simulink model "PVtestsiteeight"  (Simulink 10.1)
settings: Solver=FixedStepDiscrete  StartTime=0.0  StopTime=inf  FixedStep=Ts  RelTol=1e-3
PreLoadFcn:
  | init_DCDCDCAC_new
InitFcn:
  | init_DCDCDCAC_new
undefined symbols (not defined in the file or in its folder): D1, Delta, I, Left, Right, type, V
libraries: powerlib x174, powerlib_meascontrol x3, ssn_lib x2, artemis x1
(part 1 of 3)
settings Model: ARTEMISmethode_block_infos=$$__separator__$$PVtestsiteeight/SS_Grid/ARTEMIS Guide$$__separator__$$  Creator=jz38692  LastModifiedBy=jz38692
settings DataIOCC: ExternalInput=ILreplay  SaveFormat=Dataset  SaveOutput=off  SignalLogging=off  DSMLogging=off  SaveTime=off  DSMLoggingName=signal_recordone
settings OptimizationCC: LifeSpan=auto
settings DebuggingCC: UnderspecifiedInitializationDetection=Simplified  MergeDetectMultiDrivingBlocksExec=error  SFUnexpectedBacktrackingDiag=error  SFNoUnconditionalDefaultTransitionDiag=error  SFExecutionAtInitializationDiag=warning
settings HardwareCC: ProdBitPerPointer=64  ProdBitPerSizeT=64  ProdBitPerPtrDiffT=64  ProdLargestAtomicFloat=Float  ProdIntDivRoundTo=Zero  ProdEndianess=LittleEndian  ProdWordSize=64  ProdHWDeviceType=Intel->x86-64 (Windows64)
settings ModelReferenceCC: PropagateSignalLabelsOutOfModel=on
settings SFSimCC: SimUseLocalCustomCode=on
settings RTWCC: RTWUseLocalCustomCode=on
settings GRTTargetCC: TargetLangStandard=C99 (ISO)  CombineOutputUpdateFcns=on  GRTInterface=off
settings ConfigComp: CovMetricSettings=dwe  CovHtmlReporting=off  CovSaveCumulativeToWorkspaceVar=off  CovSaveSingleToWorkspaceVar=off  CovExternalEMLEnable=on
settings SimscapeCC: SimscapeNormalizeSystem=off

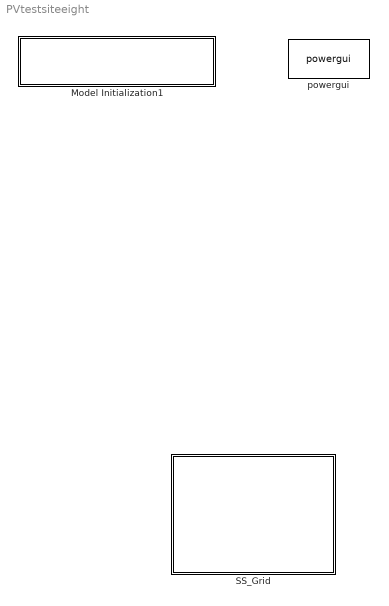
== system PVtestsiteeight ==
  Model Initialization1 : Subsystem  AncestorBlock=artemis/Tools /Misc/Model Initialization  mask(Model Functions){InitFcnX=init_DCDCDCAC_new, prel=on, posl=off, inif=on, strf=off}
      mask prompts: InitFcnX "Initialisation"; prel "Preload Function"; posl "PostLoad Function"; inif "InitFcn"; strf "StartFcn"
      mask init:
      | currentBlock = gcb;
      | root = bdroot(currentBlock);
      | 
      | if ~strcmp(get_param(root,'BlockDiagramType'),'library')
      |     if prel==1
      |         set_param(root, 'PreLoadFcn', InitFcnX);
      |     else
      |         set_param(root, 'PreLoadFcn', '');
      |     end
      |     if inif==1
      |         set_param(root, 'InitFcn', InitFcnX);
      |     else
      |         set_param(root, 'InitFcn', '');
      |     end
      |     if strf==1
      |         set_param(root, 'StartFcn', InitFcnX);
      |     else
      |         set_param(root, 'StartFcn', '');
      |     end
      |     if posl==1
      |         set_param(root, 'PostLoadFcn', InitFcnX);
      |     else
      |         set_param(root, 'PostLoadFcn', '');
      |     end
      | end
      | 
      | pos = get_param(currentBlock, 'Position');
      | width = pos(3) - pos(1); height = pos(4) - pos(2);
      | txt = [ upper(root) '\n' '- InitFcn. . . . . '  get_param(root, 'InitFcn') ];
      settings: CopyFcn=set_param(gcb,'LinkStatus','inactive')
      mask Display: text(5, height*0.5, txt, 'horizontalAlignment', 'left', 'verticalAlignment', 'middle') ;
  SS_Grid : Subsystem
  powergui : powerlib/powergui  Priority=1  SimulationMode=Discrete  SampleTime=5e-5  frequency=60  Iterations=50  frequencyindice=0  Pbase=100e6  ErrMax=1e-4  UnitsV=kV  UnitsW=MW  buscounter=0  FunctionMessages=off  echomessages=off  EnableUseOfTLC=off  CurrentSourceSwitches=off  DisableSnubberDevices=off  DisableRonSwitches=off  DisableVfSwitches=off  DisplayEquations=off  AutomaticDiscreteSolvers=off  SolverType=Backward Euler  Interpol=off  ExternalGateDelay=off  methode=off  Ts=100  x0status=blocks  SPID=off  SwTol=0  HookPort=off  NonlinearTolerance=1e-4  nMaxIteration=100  ContinueOnMaxIteration=off  RestoreLinks=warning  ResistiveCurrentMeasurement=off  Frange=[0:2:500]  Ylog=off  Xlog=on  ShowGrid=off  save=off  variable=ZData  structure=UIC  ZoomFFT=off  StartTime=1  cycles=50  DisplayStyle=1  fundamental=60  FreqAxis=off  MaxFrequency=10000  frequencyindicesteady=1  RmsSteady=1  display=off

== system PVtestsiteeight/Model Initialization1 ==

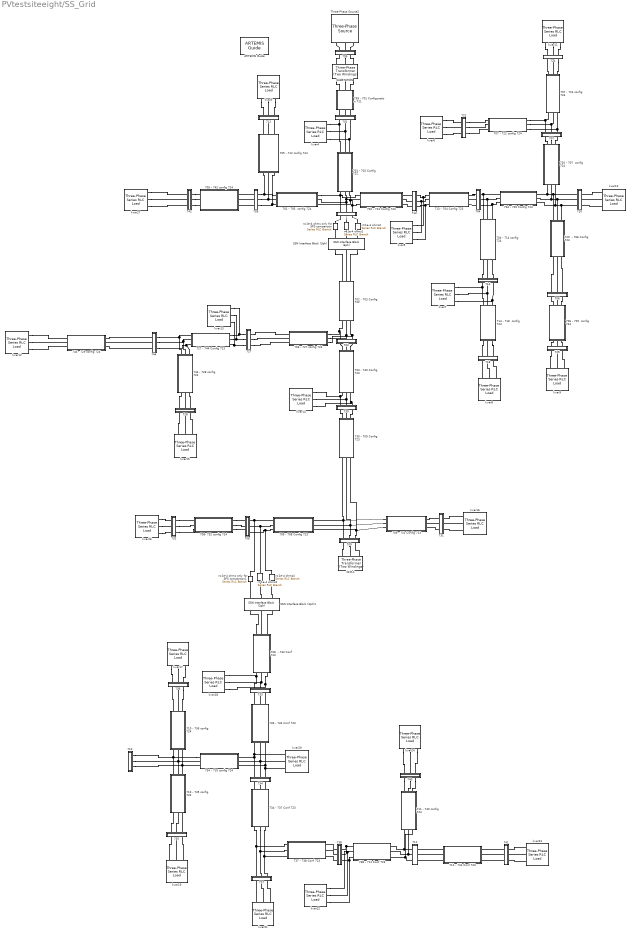
== system PVtestsiteeight/SS_Grid ==
  " 738 - 711 Conf 723 " : Subsystem  mask{D=0.1219}
      mask prompts: D "Distance (km)"
   kvar{5..11,14,16..24,26..27} (19 alike) : powerlib/Elements/Three-Phase Series RLC Load  LConnTagsString=A|B|C  Configuration=Y (grounded)  NominalVoltage=4800  Vabc=[4.8e3 4.8e3 4.8e3]/sqrt(3)  Vabcp=[1e3 1e3 1e3]  NominalFrequency=60  UnbalancedPower=on  ActivePower=10000  InductivePower=0  CapacitivePower=0  Pabc=[10e3 10e3 10e3]  QLabc=[0 0 0]  QCabc=[0 0 0]  Pabcp=[10e3 9e3 11e3]  QLabcp=[100 90 110]  QCabcp=[100 90 110]  Measurements=None  LoadType=constant Z
  " kvar12" : powerlib/Elements/Three-Phase Series RLC Load  LConnTagsString=A|B|C  Configuration=Y (grounded)  NominalVoltage=4800  Vabc=[4.8e3 4.8e3 4.8e3]/sqrt(3)  Vabcp=[1e3 1e3 1e3]  NominalFrequency=60  UnbalancedPower=off  ActivePower=100000  InductivePower=5000  CapacitivePower=0  Pabc=[10e3 10e3 10e3]  QLabc=[0 0 0]  QCabc=[0 0 0]  Pabcp=[10e3 9e3 11e3]  QLabcp=[100 90 110]  QCabcp=[100 90 110]  Measurements=None  LoadType=constant Z
  " kvar13" : powerlib/Elements/Three-Phase Series RLC Load  LConnTagsString=A|B|C  Configuration=Y (grounded)  NominalVoltage=4800  Vabc=[4.8e3 4.8e3 4.8e3]/sqrt(3)  Vabcp=[1e3 1e3 1e3]  NominalFrequency=60  UnbalancedPower=off  ActivePower=200000  InductivePower=5000  CapacitivePower=0  Pabc=[10e3 10e3 10e3]  QLabc=[0 0 0]  QCabc=[0 0 0]  Pabcp=[10e3 9e3 11e3]  QLabcp=[100 90 110]  QCabcp=[100 90 110]  Measurements=None  LoadType=constant Z
  " kvar15" : powerlib/Elements/Three-Phase Series RLC Load  LConnTagsString=A|B|C  Configuration=Y (grounded)  NominalVoltage=4800  Vabc=[4.8e3 4.8e3 4.8e3]/sqrt(3)  Vabcp=[1e3 1e3 1e3]  NominalFrequency=60  UnbalancedPower=off  ActivePower=200000  InductivePower=5000  CapacitivePower=0  Pabc=[10e3 10e3 10e3]  QLabc=[0 0 0]  QCabc=[0 0 0]  Pabcp=[10e3 9e3 11e3]  QLabcp=[100 90 110]  QCabcp=[100 90 110]  Measurements=None  LoadType=constant Z
  " kvar3" : powerlib/Elements/Three-Phase Series RLC Load  LConnTagsString=A|B|C  Configuration=Y (grounded)  NominalVoltage=4800  Vabc=[4.8e3 4.8e3 4.8e3]/sqrt(3)  Vabcp=[1e3 1e3 1e3]  NominalFrequency=60  UnbalancedPower=on  ActivePower=10000  InductivePower=0  CapacitivePower=0  Pabc=[3e3 3e3 3e3]  QLabc=[0 0 0]  QCabc=[0 0 0]  Pabcp=[10e3 9e3 11e3]  QLabcp=[100 90 110]  QCabcp=[100 90 110]  Measurements=None  LoadType=constant Z
  " kvar4" : powerlib/Elements/Three-Phase Series RLC Load  LConnTagsString=A|B|C  Configuration=Y (grounded)  NominalVoltage=4800  Vabc=[4.8e3 4.8e3 4.8e3]  Vabcp=[1e3 1e3 1e3]  NominalFrequency=60  UnbalancedPower=on  ActivePower=10000  InductivePower=0  CapacitivePower=0  Pabc=[3e3 3e3 3e3]  QLabc=[100 100 100]  QCabc=[0 0 0]  Pabcp=[10e3 9e3 11e3]  QLabcp=[100 90 110]  QCabcp=[100 90 110]  Measurements=None  LoadType=constant Z
  1 : Subsystem  mask{I=I_702, V=V_702}
      mask prompts: I "Current"; V "Voltage"
      mask TypeOptions I: Goto/GotoTag
      mask TypeOptions V: Goto1/GotoTag
      mask Display: text(10,20, 'ABC')
  701 : Subsystem  mask{I=I_701, V=V_701}
      mask prompts: I "Current"; V "Voltage"
      mask TypeOptions I: Goto/GotoTag
      mask TypeOptions V: Goto1/GotoTag
      mask Display: text(10,20, 'ABC')
  701 - 702 Config 722 : Subsystem  mask{D=0.2926}
      mask prompts: D "Distance (km)"
  702 - 703 Config 722 : Subsystem  mask{D=0.4023}
      mask prompts: D "Distance (km)"
  "702 - 705  config 724 " : Subsystem  mask{D=0.1219}
      mask prompts: D "Distance (km)"
  702 - 713 Config 723 : Subsystem  mask{D=0.1097}
      mask prompts: D "Distance (km)"
  703 : Subsystem  mask{I=I_703, V=V_703}
      mask prompts: I "Current"; V "Voltage"
      mask TypeOptions I: Goto/GotoTag
      mask TypeOptions V: Goto1/GotoTag
      mask Display: text(10,20, 'ABC')
  703 - 727 config 724 : Subsystem  mask{D=0.0732}
      mask prompts: D "Distance (km)"
  703 - 730 Config 723 : Subsystem  mask{D=0.1829}
      mask prompts: D "Distance (km)"
  704 : Subsystem  mask{I=I_704, V=V_704}
      mask prompts: I "Current"; V "Voltage"
      mask TypeOptions I: Goto/GotoTag
      mask TypeOptions V: Goto1/GotoTag
      mask Display: text(10,20, 'ABC')
  704 - 714 config 724 : Subsystem  mask{D=0.0244}
      mask prompts: D "Distance (km)"
  704 - 720 Config 723 : Subsystem  mask{D=0.2438}
      mask prompts: D "Distance (km)"
  705 : Subsystem  mask{I=I_705, V=V_705}
      mask prompts: I "Current"; V "Voltage"
      mask TypeOptions I: Goto/GotoTag
      mask TypeOptions V: Goto1/GotoTag
      mask Display: text(10,20, 'ABC')
  "705 - 712 config 724 " : Subsystem  mask{D=0.0732}
      mask prompts: D "Distance (km)"
  705 - 742 config 724 : Subsystem  mask{D=0.0975}
      mask prompts: D "Distance (km)"
  706 : Subsystem  mask{I=I_706, V=V_706}
      mask prompts: I "Current"; V "Voltage"
      mask TypeOptions I: Goto/GotoTag
      mask TypeOptions V: Goto1/GotoTag
      mask Display: text(10,20, 'ABC')
  706 - 725  config 724 : Subsystem  mask{D=0.0853}
      mask prompts: D "Distance (km)"
  707 : Subsystem  mask{I=I_707, V=V_707}
      mask prompts: I "Current"; V "Voltage"
      mask TypeOptions I: Goto/GotoTag
      mask TypeOptions V: Goto1/GotoTag
      mask Display: text(10,20, 'ABC')
  707 - 722 config 724 : Subsystem  mask{D=0.0366}
      mask prompts: D "Distance (km)"
  707 - 724 config 724 : Subsystem  mask{D=0.2316}
      mask prompts: D "Distance (km)"
  708 : Subsystem  mask{I=I_708, V=V_708}
      mask prompts: I "Current"; V "Voltage"
      mask TypeOptions I: Goto/GotoTag
      mask TypeOptions V: Goto1/GotoTag
      mask Display: text(10,20, 'ABC')
  708  - 733 Conf 723 : Subsystem  mask{D=0.0975}
      mask prompts: D "Distance (km)"
  "708- 732 config 724 " : Subsystem  mask{D=0.0975}
      mask prompts: D "Distance (km)"
  709 : Subsystem  mask{I=I_709, V=V_709}
      mask prompts: I "Current"; V "Voltage"
      mask TypeOptions I: Goto/GotoTag
      mask TypeOptions V: Goto1/GotoTag
      mask Display: text(10,20, 'ABC')
  709 - 708 Config 723 : Subsystem  mask{D=0.0975}
      mask prompts: D "Distance (km)"
  709 - 731 Config 723 : Subsystem  mask{D=0.1829}
      mask prompts: D "Distance (km)"
  710 : Subsystem  mask{I=I_710, V=V_710}
      mask prompts: I "Current"; V "Voltage"
      mask TypeOptions I: Goto/GotoTag
      mask TypeOptions V: Goto1/GotoTag
      mask Display: text(10,20, 'ABC')
  "710 - 735 config 724 " : Subsystem  mask{D=0.061}
      mask prompts: D "Distance (km)"
  "710 - 736 config 724 " : Subsystem  mask{D=0.3901}
      mask prompts: D "Distance (km)"
  711 : Subsystem  mask{I=I_711, V=V_711}
      mask prompts: I "Current"; V "Voltage"
      mask TypeOptions I: Goto/GotoTag
      mask TypeOptions V: Goto1/GotoTag
      mask Display: text(10,20, 'ABC')
  "711 - 740 config 724 " : Subsystem  mask{D=0.061}
      mask prompts: D "Distance (km)"
  "711 - 741 Conf 723 " : Subsystem  mask{D=0.1219}
      mask prompts: D "Distance (km)"
  712 : Subsystem  mask{I=I_712, V=V_712}
      mask prompts: I "Current"; V "Voltage"
      mask TypeOptions I: Goto/GotoTag
      mask TypeOptions V: Goto1/GotoTag
      mask Display: text(10,20, 'ABC')
  713 : Subsystem  mask{I=I_713, V=V_713}
      mask prompts: I "Current"; V "Voltage"
      mask TypeOptions I: Goto/GotoTag
      mask TypeOptions V: Goto1/GotoTag
      mask Display: text(10,20, 'ABC')
  713 - 704 Config 723 : Subsystem  mask{D=0.1585}
      mask prompts: D "Distance (km)"
  714 : Subsystem  mask{I=I_714, V=V_714}
      mask prompts: I "Current"; V "Voltage"
      mask TypeOptions I: Goto/GotoTag
      mask TypeOptions V: Goto1/GotoTag
      mask Display: text(10,20, 'ABC')
  714 - 718  config 724 : Subsystem  mask{D=0.1585}
      mask prompts: D "Distance (km)"
  718 : Subsystem  mask{I=I_718, V=V_718}
      mask prompts: I "Current"; V "Voltage"
      mask TypeOptions I: Goto/GotoTag
      mask TypeOptions V: Goto1/GotoTag
      mask Display: text(10,20, 'ABC')
  720 : Subsystem  mask{I=I_720, V=V_720}
      mask prompts: I "Current"; V "Voltage"
      mask TypeOptions I: Goto/GotoTag
      mask TypeOptions V: Goto1/GotoTag
      mask Display: text(10,20, 'ABC')
  720  - 706 Config 723 : Subsystem  mask{D=0.1829}
      mask prompts: D "Distance (km)"
  720 - 707  config 724 : Subsystem  mask{D=0.2804}
      mask prompts: D "Distance (km)"
  722 : Subsystem  mask{I=I_722, V=V_722}
      mask prompts: I "Current"; V "Voltage"
      mask TypeOptions I: Goto/GotoTag
      mask TypeOptions V: Goto1/GotoTag
      mask Display: text(10,20, 'ABC')
  724 : Subsystem  mask{I=I_724, V=V_724}
      mask prompts: I "Current"; V "Voltage"
      mask TypeOptions I: Goto/GotoTag
      mask TypeOptions V: Goto1/GotoTag
      mask Display: text(10,20, 'ABC')
  725 : Subsystem  mask{I=I_725, V=V_725}
      mask prompts: I "Current"; V "Voltage"
      mask TypeOptions I: Goto/GotoTag
      mask TypeOptions V: Goto1/GotoTag
      mask Display: text(10,20, 'ABC')
  727 : Subsystem  mask{I=I_727, V=V_727}
      mask prompts: I "Current"; V "Voltage"
      mask TypeOptions I: Goto/GotoTag
      mask TypeOptions V: Goto1/GotoTag
      mask Display: text(10,20, 'ABC')
  727 - 744 Config 723 : Subsystem  mask{D=0.0853}
      mask prompts: D "Distance (km)"
  728 : Subsystem  mask{I=I_728, V=V_728}
      mask prompts: I "Current"; V "Voltage"
      mask TypeOptions I: Goto/GotoTag
      mask TypeOptions V: Goto1/GotoTag
      mask Display: text(10,20, 'ABC')
  730 : Subsystem  mask{I=I_730, V=V_730}
      mask prompts: I "Current"; V "Voltage"
      mask TypeOptions I: Goto/GotoTag
      mask TypeOptions V: Goto1/GotoTag
      mask Display: text(10,20, 'ABC')
  730 - 709 Config 723 : Subsystem  mask{D=0.061}
      mask prompts: D "Distance (km)"
  731 : Subsystem  mask{I=I_731, V=V_731}
      mask prompts: I "Current"; V "Voltage"
      mask TypeOptions I: Goto/GotoTag
      mask TypeOptions V: Goto1/GotoTag
      mask Display: text(10,20, 'ABC')
  732 : Subsystem  mask{I=I_732, V=V_732}
      mask prompts: I "Current"; V "Voltage"
      mask TypeOptions I: Goto/GotoTag
      mask TypeOptions V: Goto1/GotoTag
      mask Display: text(10,20, 'ABC')
  733 : Subsystem  mask{I=I_733, V=V_733}
      mask prompts: I "Current"; V "Voltage"
      mask TypeOptions I: Goto/GotoTag
      mask TypeOptions V: Goto1/GotoTag
      mask Display: text(10,20, 'ABC')
  733 - 734 Conf 723 : Subsystem  mask{D=0.1707}
      mask prompts: D "Distance (km)"
  734 : Subsystem  mask{I=I_734, V=V_734}
      mask prompts: I "Current"; V "Voltage"
      mask TypeOptions I: Goto/GotoTag
      mask TypeOptions V: Goto1/GotoTag
      mask Display: text(10,20, 'ABC')
  "734 - 710 config 724 " : Subsystem  mask{D=0.1585}
      mask prompts: D "Distance (km)"
  "734 - 737 Conf 723 " : Subsystem  mask{D=0.1951}
      mask prompts: D "Distance (km)"
  735 : Subsystem  mask{I=I_735, V=V_735}
      mask prompts: I "Current"; V "Voltage"
      mask TypeOptions I: Goto/GotoTag
      mask TypeOptions V: Goto1/GotoTag
      mask Display: text(10,20, 'ABC')
  736 : Subsystem  mask{I=I_736, V=V_736}
      mask prompts: I "Current"; V "Voltage"
      mask TypeOptions I: Goto/GotoTag
      mask TypeOptions V: Goto1/GotoTag
      mask Display: text(10,20, 'ABC')
  737 : Subsystem  mask{I=I_737, V=V_737}
      mask prompts: I "Current"; V "Voltage"
      mask TypeOptions I: Goto/GotoTag
      mask TypeOptions V: Goto1/GotoTag
      mask Display: text(10,20, 'ABC')
  "737 - 738 Conf 723 " : Subsystem  mask{D=0.1219}
      mask prompts: D "Distance (km)"
  738 : Subsystem  mask{I=I_738, V=V_738}
      mask prompts: I "Current"; V "Voltage"
      mask TypeOptions I: Goto/GotoTag
      mask TypeOptions V: Goto1/GotoTag
      mask Display: text(10,20, 'ABC')
  740 : Subsystem  mask{I=I_740, V=V_740}
      mask prompts: I "Current"; V "Voltage"
      mask TypeOptions I: Goto/GotoTag
      mask TypeOptions V: Goto1/GotoTag
      mask Display: text(10,20, 'ABC')
  741 : Subsystem  mask{I=I_741, V=V_741}
      mask prompts: I "Current"; V "Voltage"
      mask TypeOptions I: Goto/GotoTag
      mask TypeOptions V: Goto1/GotoTag
      mask Display: text(10,20, 'ABC')
  742 : Subsystem  mask{I=I_742, V=V_742}
      mask prompts: I "Current"; V "Voltage"
      mask TypeOptions I: Goto/GotoTag
      mask TypeOptions V: Goto1/GotoTag
      mask Display: text(10,20, 'ABC')
  744 : Subsystem  mask{I=I_744, V=V_744}
      mask prompts: I "Current"; V "Voltage"
      mask TypeOptions I: Goto/GotoTag
      mask TypeOptions V: Goto1/GotoTag
      mask Display: text(10,20, 'ABC')
  "744 - 728 config 724 " : Subsystem  mask{D=0.0610}
      mask prompts: D "Distance (km)"
  "744 - 729 config 724 " : Subsystem  mask{D=0.0853}
      mask prompts: D "Distance (km)"
  799 : Subsystem  mask{I=I_799, V=V_799}
      mask prompts: I "Current"; V "Voltage"
      mask TypeOptions I: Goto/GotoTag
      mask TypeOptions V: Goto1/GotoTag
      mask Display: text(10,20, 'ABC')
  799 - 701 Configuration 721 : Subsystem  mask{D=0.5639}
      mask prompts: D "Distance (km)"
  ARTEMIS Guide : artemis/ARTEMIS/ARTEMIS Guide  Tag=FTSSmethode_opal_4hx0r99  Description=5.0_z1  lock=on  Ts=5e-5  opt=art5  dyna=off  nb_perm=4  RT_fullcomp=off  ssn=on  ssn_itvc=off  ssn_ivic=off  ssn_ext=off  ssn_solver=Art5  ssn_impulse=off  ssn_quasimpulse=off  ssn_impulse_loop=2  paraExtinctionThy=off  Thy_Impulse=on  dtc=Off  dtc_opt=normal  ao=on  simtype=off  ct_mac=off  lin_mov=off  lsp=[0.001 2]  spike_skip=Disabled  dtc_extra=1  dtc_sws=normal  dtc_pied=0.5  SPSRulesBlock=SPSRules  tre=on  ctmm=off  LF=off  dpl_type=ARTEMiS DPL  rlc_type=off  custom_type=off  para=on  ssn_ImpulseLoopBlockedStateUpdate=2  ssn_mov_iter_number=5  ssn_switch_iter_number=5  ssn_nib_type_verify=on  ssn_use_lu=on  ssn_use_ldlt=off  ssn_full_iteration=off
  SSN Interface Block (3ph) : ssn_lib/SSN Interface Block (3ph)  nb_phase=3  nb_port=2  p1_type=I-type(Left)  p2_type=I-type(Right)  p3_type=V-type(Left)  p4_type=V-type(Left)  p5_type=V-type(Left)  p6_type=V-type(Left)  p7_type=V-type(Left)  p8_type=V-type(Left)  p9_type=V-type(Left)  p10_type=V-type(Left)  p11_type=V-type(Left)  p12_type=V-type(Left)  p13_type=V-type(Left)  p14_type=V-type(Left)  p15_type=V-type(Left)  p16_type=V-type(Left)  I_port_shunt_resistance=1e9
  SSN Interface Block (3ph)1 : ssn_lib/SSN Interface Block (3ph)  nb_phase=3  nb_port=2  p1_type=I-type(Left)  p2_type=I-type(Right)  p3_type=V-type(Left)  p4_type=V-type(Left)  p5_type=V-type(Left)  p6_type=V-type(Left)  p7_type=V-type(Left)  p8_type=V-type(Left)  p9_type=V-type(Left)  p10_type=V-type(Left)  p11_type=V-type(Left)  p12_type=V-type(Left)  p13_type=V-type(Left)  p14_type=V-type(Left)  p15_type=V-type(Left)  p16_type=V-type(Left)  I_port_shunt_resistance=1e9
  SUBSTATION : powerlib/Elements/Three-Phase Transformer (Two Windings)  Winding1Connection=Yg  Winding2Connection=Yg  CoreType=Three single-phase transformers  SetSaturation=off  Hysteresis=off  DataFile='hysteresis'  SetInitialFlux=off  Measurements=None  UNITS=pu  NominalPower=[ 2500e3 , 60 ]  Winding1=[ 230e3 , 0.01 , 0.04 ]  Winding2=[ 4.8e3 , 0.01 , 0.04 ]  Rm=500  Lm=500  L0=0.5  Saturation=[ 0,0 ; 0.0024,1.2 ; 1.0,1.52 ]  InitialFluxes=[ 0.8 , -0.8 , 0.7 ]  BreakLoop=off  DiscreteSolver=Trapezoidal iterative  DataType=off  TransfoNumber=1
  Three-Phase Source2 : powerlib/Electrical Sources/Three-Phase Source  InternalConnection=Yg  VoltagePhases=off  Voltage=230e3  PhaseAngle=0  Voltage_phases=[25e3 25e3 25e3]/sqrt(3)  PhaseAngles_phases=[0 -120 +120]  Frequency=60  NonIdealSource=on  SpecifyImpedance=on  Resistance=0.8929  Inductance=16.58e-3  ShortCircuitLevel=100e6  BaseVoltage=230e3  XRratio=7  BusType=swing  Pref=inf  Qref=inf  Prefabc=[10e3, 10e3, 10e3]  Qrefabc=[0, 0, 0]  Qmin=-inf  Qmax=inf
  XFM-1 : powerlib/Elements/Three-Phase Transformer (Two Windings)  Winding1Connection=Delta (D1)  Winding2Connection=Delta (D1)  CoreType=Three single-phase transformers  SetSaturation=off  Hysteresis=off  DataFile='hysteresis'  SetInitialFlux=off  Measurements=None  UNITS=pu  NominalPower=[ 500e3 , 60 ]  Winding1=[ 4.8e3 , 0.00045 , 0.00905 ]  Winding2=[ 0.48e3 , 0.00045 , 0.00905 ]  Rm=500  Lm=500  L0=0.5  Saturation=[ 0,0 ; 0.0024,1.2 ; 1.0,1.52 ]  InitialFluxes=[ 0.8 , -0.8 , 0.7 ]  BreakLoop=off  DiscreteSolver=Trapezoidal iterative  DataType=off  TransfoNumber=1
  r=1e-4 ohms only for SPS comparison : powerlib/Elements/Series RLC Branch  LConnTagsString=__new0  RConnTagsString=__new0  BranchType=R  Resistance=1e-4  Inductance=1e-3  SetiL0=off  InitialCurrent=0  Capacitance=1e-6  Setx0=off  InitialVoltage=0  Measurements=None
  r=1e-4 ohms only for SPS comparison1 : powerlib/Elements/Series RLC Branch  LConnTagsString=__new0  RConnTagsString=__new0  BranchType=R  Resistance=1e-4  Inductance=1e-3  SetiL0=off  InitialCurrent=0  Capacitance=1e-6  Setx0=off  InitialVoltage=0  Measurements=None
  r=1e-4 ohms{1..4} (4 alike) : powerlib/Elements/Series RLC Branch  LConnTagsString=__new0  RConnTagsString=__new0  BranchType=R  Resistance=1e-4  Inductance=1e-3  SetiL0=off  InitialCurrent=0  Capacitance=1e-6  Setx0=off  InitialVoltage=0  Measurements=None
  connections:
  "702 - 705  config 724 "/RConn3 -- 701 - 702 Config 722/LConn3 -- 702 - 713 Config 723/LConn3 -- 1/LConn3
  1/LConn2 -- "702 - 705  config 724 "/RConn2 -- 701 - 702 Config 722/LConn2 -- 702 - 713 Config 723/LConn2
  702 - 703 Config 722/LConn3 -- 703/RConn3 -- 703 - 727 config 724/RConn3
  703 - 727 config 724/RConn2 -- 703/RConn2 -- 702 - 703 Config 722/LConn2
  703 - 727 config 724/RConn1 -- 703/RConn1 -- 702 - 703 Config 722/LConn1
  709/RConn2 -- 709 - 731 Config 723/LConn2 -- 709 - 708 Config 723/RConn2 -- 730 - 709 Config 723/LConn2
  709/RConn1 -- 709 - 731 Config 723/LConn1 -- 709 - 708 Config 723/RConn1 -- 730 - 709 Config 723/LConn1
  709/RConn3 -- 709 - 731 Config 723/LConn3 -- 709 - 708 Config 723/RConn3 -- 730 - 709 Config 723/LConn3
  "705 - 712 config 724 "/RConn3 -- 705/RConn3 -- "702 - 705  config 724 "/LConn3
  705/RConn2 -- "702 - 705  config 724 "/LConn2 -- "705 - 712 config 724 "/RConn2
  "702 - 705  config 724 "/LConn1 -- 705/RConn1 -- "705 - 712 config 724 "/RConn1
  "744 - 728 config 724 "/LConn1 -- 744/RConn1 -- 727 - 744 Config 723/LConn1
  "744 - 728 config 724 "/LConn2 -- 744/RConn2 -- 727 - 744 Config 723/LConn2
  "744 - 728 config 724 "/LConn3 -- 744/RConn3 -- 727 - 744 Config 723/LConn3
  704 - 714 config 724/LConn3 -- 704/RConn3 -- 704 - 720 Config 723/LConn3
  704 - 714 config 724/LConn2 -- 704/RConn2 -- 704 - 720 Config 723/LConn2
  704 - 720 Config 723/LConn1 -- 704 - 714 config 724/LConn1 -- 704/RConn1
  704 - 720 Config 723/RConn3 -- 720 - 707  config 724/RConn3 -- 720  - 706 Config 723/RConn3 -- 720/LConn3
  704 - 720 Config 723/RConn2 -- 720 - 707  config 724/RConn2 -- 720/LConn2 -- 720  - 706 Config 723/RConn2
  704 - 720 Config 723/RConn1 -- 720 - 707  config 724/RConn1 -- 720  - 706 Config 723/RConn1 -- 720/LConn1
  707 - 722 config 724/RConn3 -- 707/LConn3 -- 707 - 724 config 724/RConn3
  707 - 722 config 724/RConn2 -- 707/LConn2 -- 707 - 724 config 724/RConn2
  707 - 722 config 724/RConn1 -- 707/LConn1 -- 707 - 724 config 724/RConn1
  709 - 708 Config 723/LConn3 -- 708/RConn3 -- r=1e-4 ohms4/LConn1
  709 - 708 Config 723/LConn2 -- 708/RConn2 -- r=1e-4 ohms3/LConn1
  709 - 708 Config 723/LConn1 -- 708/RConn1 -- r=1e-4 ohms only for SPS comparison1/LConn1
  "734 - 710 config 724 "/RConn3 -- 733 - 734 Conf 723/LConn3 -- " kvar20"/LConn3 -- 734/LConn3
  733 - 734 Conf 723/LConn2 -- 734/LConn2 -- " kvar20"/LConn2 -- "734 - 710 config 724 "/RConn2
  734/LConn1 -- "734 - 710 config 724 "/RConn1 -- " kvar20"/LConn1 -- 733 - 734 Conf 723/LConn1
  710/LConn3 -- "710 - 736 config 724 "/RConn3 -- "734 - 710 config 724 "/LConn3 -- "710 - 735 config 724 "/LConn3
  710/LConn2 -- "710 - 736 config 724 "/RConn2 -- "734 - 710 config 724 "/LConn2 -- "710 - 735 config 724 "/LConn2
  "734 - 710 config 724 "/LConn1 -- "710 - 735 config 724 "/LConn1 -- "710 - 736 config 724 "/RConn1 -- 710/LConn1
  "734 - 737 Conf 723 "/LConn1 -- "737 - 738 Conf 723 "/LConn1 -- 737/LConn1
  "734 - 737 Conf 723 "/LConn2 -- "737 - 738 Conf 723 "/LConn2 -- 737/LConn2
  "737 - 738 Conf 723 "/LConn3 -- 737/LConn3 -- "734 - 737 Conf 723 "/LConn3
  " 738 - 711 Conf 723 "/RConn3 -- 711/RConn3 -- "711 - 740 config 724 "/RConn3
  " 738 - 711 Conf 723 "/RConn2 -- 711/RConn2 -- "711 - 740 config 724 "/RConn2
  " 738 - 711 Conf 723 "/RConn1 -- 711/RConn1 -- "711 - 740 config 724 "/RConn1
  701 - 702 Config 722/LConn1 -- 702 - 713 Config 723/LConn1 -- 1/LConn1 -- "702 - 705  config 724 "/RConn1
  714/RConn2 -- 714 - 718  config 724/LConn2 -- " kvar7"/LConn2
  701/LConn1 -- 701 - 702 Config 722/RConn1 -- " kvar4"/LConn1
  " kvar7"/LConn1 -- 714 - 718  config 724/LConn1 -- 714/RConn1
  713 - 704 Config 723/LConn1 -- 713/RConn1 -- " kvar5"/LConn1
  701/LConn2 -- 701 - 702 Config 722/RConn2 -- " kvar4"/LConn2
  714/RConn3 -- 714 - 718  config 724/LConn3 -- " kvar7"/LConn3
  713 - 704 Config 723/LConn3 -- 713/RConn3 -- " kvar5"/LConn3
  " kvar4"/LConn3 -- 701 - 702 Config 722/RConn3 -- 701/LConn3
  738/LConn2 -- " 738 - 711 Conf 723 "/LConn2 -- " kvar22"/LConn2
  708  - 733 Conf 723/LConn2 -- 733/LConn2 -- " kvar18"/LConn2
  708  - 733 Conf 723/LConn1 -- 733/LConn1 -- " kvar18"/LConn1
  738/LConn1 -- " 738 - 711 Conf 723 "/LConn1 -- " kvar22"/LConn1
  703 - 730 Config 723/LConn3 -- 730/RConn3 -- " kvar14"/LConn3
  706/LConn3 -- 720  - 706 Config 723/LConn3
  " kvar14"/LConn1 -- 730/RConn1 -- 703 - 730 Config 723/LConn1
  703 - 730 Config 723/LConn2 -- 730/RConn2 -- " kvar14"/LConn2
  744/LConn3 -- "744 - 729 config 724 "/RConn3
  727/LConn1 -- 727 - 744 Config 723/RConn1 -- " kvar13"/LConn1
  727/LConn2 -- 727 - 744 Config 723/RConn2 -- " kvar13"/LConn2
  744/LConn2 -- "744 - 729 config 724 "/RConn2
  744/LConn1 -- "744 - 729 config 724 "/RConn1
  706/LConn2 -- 720  - 706 Config 723/LConn2
  713 - 704 Config 723/LConn2 -- 713/RConn2 -- " kvar5"/LConn2
  738/LConn3 -- " 738 - 711 Conf 723 "/LConn3 -- " kvar22"/LConn3
  708  - 733 Conf 723/LConn3 -- 733/LConn3 -- " kvar18"/LConn3
  727/LConn3 -- 727 - 744 Config 723/RConn3 -- " kvar13"/LConn3
  706/LConn1 -- 720  - 706 Config 723/LConn1
  727/RConn2 -- 703 - 727 config 724/LConn2
  727/RConn1 -- 703 - 727 config 724/LConn1
  727/RConn3 -- 703 - 727 config 724/LConn3
  799/RConn1 -- Three-Phase Source2/RConn1
  799/LConn1 -- SUBSTATION/LConn1
  707/RConn1 -- 720 - 707  config 724/LConn1
  706 - 725  config 724/LConn3 -- 706/RConn3
  740/LConn3 -- "711 - 740 config 724 "/LConn3
  799/LConn3 -- SUBSTATION/LConn3
  705/LConn2 -- 705 - 742 config 724/LConn2
  SSN Interface Block (3ph)1/LConn1 -- r=1e-4 ohms only for SPS comparison1/RConn1
  SSN Interface Block (3ph)/LConn1 -- r=1e-4 ohms only for SPS comparison/RConn1
  r=1e-4 ohms1/LConn1 -- 1/RConn2
  SSN Interface Block (3ph)1/LConn3 -- r=1e-4 ohms4/RConn1
  "710 - 736 config 724 "/LConn1 -- 736/RConn1
  799/RConn3 -- Three-Phase Source2/RConn3
  735/LConn1 -- "710 - 735 config 724 "/RConn1
  SSN Interface Block (3ph)/LConn3 -- r=1e-4 ohms2/RConn1
  799/RConn2 -- Three-Phase Source2/RConn2
  SSN Interface Block (3ph)/RConn1 -- 702 - 703 Config 722/RConn1
  728/LConn2 -- "744 - 728 config 724 "/RConn2
  703 - 730 Config 723/RConn3 -- 703/LConn3
  SSN Interface Block (3ph)/RConn3 -- 702 - 703 Config 722/RConn3
  701/RConn2 -- 799 - 701 Configuration 721/RConn2
  742/RConn2 -- 705 - 742 config 724/RConn2
  "708- 732 config 724 "/RConn2 -- 708/LConn2
  708  - 733 Conf 723/RConn2 -- SSN Interface Block (3ph)1/RConn2
  730/LConn3 -- 730 - 709 Config 723/RConn3
  742/RConn1 -- 705 - 742 config 724/RConn1
  705/LConn1 -- 705 - 742 config 724/LConn1
  XFM-1/LConn1 -- 709/LConn1
  "705 - 712 config 724 "/LConn3 -- 712/RConn3
  736/RConn3 -- "710 - 736 config 724 "/LConn3
  r=1e-4 ohms2/LConn1 -- 1/RConn3
  705/LConn3 -- 705 - 742 config 724/LConn3
  728/LConn3 -- "744 - 728 config 724 "/RConn3
  714 - 718  config 724/RConn3 -- 718/LConn3
  708  - 733 Conf 723/RConn1 -- SSN Interface Block (3ph)1/RConn1
  741/RConn3 -- "711 - 741 Conf 723 "/RConn3
  "705 - 712 config 724 "/LConn2 -- 712/RConn2
  " kvar6"/LConn3 -- 722/RConn3
  701/RConn1 -- 799 - 701 Configuration 721/RConn1
  SSN Interface Block (3ph)/LConn2 -- r=1e-4 ohms1/RConn1
  742/RConn3 -- 705 - 742 config 724/RConn3
  "705 - 712 config 724 "/LConn1 -- 712/RConn1
  725/LConn1 -- 706 - 725  config 724/RConn1
  799/LConn2 -- SUBSTATION/LConn2
  724/RConn2 -- 707 - 724 config 724/LConn2
  730 - 709 Config 723/RConn2 -- 730/LConn2
  "711 - 741 Conf 723 "/LConn3 -- 711/LConn3
  740/LConn1 -- "711 - 740 config 724 "/LConn1
  702 - 703 Config 722/RConn2 -- SSN Interface Block (3ph)/RConn2
  XFM-1/LConn3 -- 709/LConn3
  SSN Interface Block (3ph)1/LConn2 -- r=1e-4 ohms3/RConn1
  738/RConn1 -- "737 - 738 Conf 723 "/RConn1
  732/RConn1 -- "708- 732 config 724 "/LConn1
  736/RConn2 -- "710 - 736 config 724 "/LConn2
  707/RConn3 -- 720 - 707  config 724/LConn3
  "734 - 737 Conf 723 "/RConn1 -- 734/RConn1
  "708- 732 config 724 "/RConn3 -- 708/LConn3
  706 - 725  config 724/LConn1 -- 706/RConn1
  722/LConn1 -- 707 - 722 config 724/LConn1
  709 - 731 Config 723/RConn1 -- 731/LConn1
  738/RConn3 -- "737 - 738 Conf 723 "/RConn3
  722/LConn2 -- 707 - 722 config 724/LConn2
  703 - 730 Config 723/RConn2 -- 703/LConn2
  704/LConn1 -- 713 - 704 Config 723/RConn1
  704/LConn3 -- 713 - 704 Config 723/RConn3
  732/RConn3 -- "708- 732 config 724 "/LConn3
  704/LConn2 -- 713 - 704 Config 723/RConn2
  "711 - 741 Conf 723 "/LConn1 -- 711/LConn1
  " kvar17"/LConn3 -- 736/LConn3
  738/RConn2 -- "737 - 738 Conf 723 "/RConn2
  740/LConn2 -- "711 - 740 config 724 "/LConn2
  "734 - 737 Conf 723 "/RConn3 -- 734/RConn3
  " kvar17"/LConn1 -- 736/LConn1
  707/RConn2 -- 720 - 707  config 724/LConn2
  703 - 730 Config 723/RConn1 -- 703/LConn1
  725/LConn2 -- 706 - 725  config 724/RConn2
  713/LConn2 -- 702 - 713 Config 723/RConn2
  728/LConn1 -- "744 - 728 config 724 "/RConn1
  731/LConn3 -- 709 - 731 Config 723/RConn3
  708  - 733 Conf 723/RConn3 -- SSN Interface Block (3ph)1/RConn3
  741/RConn2 -- "711 - 741 Conf 723 "/RConn2
  701/RConn3 -- 799 - 701 Configuration 721/RConn3
  XFM-1/LConn2 -- 709/LConn2
  706 - 725  config 724/LConn2 -- 706/RConn2
  724/RConn3 -- 707 - 724 config 724/LConn3
  714/LConn2 -- 704 - 714 config 724/RConn2
  733 - 734 Conf 723/RConn2 -- 733/RConn2
  718/LConn2 -- 714 - 718  config 724/RConn2
  713/LConn1 -- 702 - 713 Config 723/RConn1
  713/LConn3 -- 702 - 713 Config 723/RConn3
  731/LConn2 -- 709 - 731 Config 723/RConn2
  "734 - 737 Conf 723 "/RConn2 -- 734/RConn2
  714/LConn1 -- 704 - 714 config 724/RConn1
  "711 - 741 Conf 723 "/LConn2 -- 711/LConn2
  733 - 734 Conf 723/RConn1 -- 733/RConn1
  722/LConn3 -- 707 - 722 config 724/LConn3
  741/RConn1 -- "711 - 741 Conf 723 "/RConn1
  1/RConn1 -- r=1e-4 ohms only for SPS comparison/LConn1
  "708- 732 config 724 "/RConn1 -- 708/LConn1
  707 - 724 config 724/LConn1 -- 724/RConn1
  733 - 734 Conf 723/RConn3 -- 733/RConn3
  " kvar3"/LConn2 -- 712/LConn2
  714/LConn3 -- 704 - 714 config 724/RConn3
  735/LConn2 -- "710 - 735 config 724 "/RConn2
  718/LConn1 -- 714 - 718  config 724/RConn1
  730/LConn1 -- 730 - 709 Config 723/RConn1
  735/LConn3 -- "710 - 735 config 724 "/RConn3
  732/RConn2 -- "708- 732 config 724 "/LConn2
  725/LConn3 -- 706 - 725  config 724/RConn3
  " kvar9"/LConn3 -- 725/RConn3
  SUBSTATION/RConn3 -- 799 - 701 Configuration 721/LConn3
  SUBSTATION/RConn2 -- 799 - 701 Configuration 721/LConn2
  " kvar17"/LConn2 -- 736/LConn2
  " kvar8"/LConn3 -- 718/RConn3
  " kvar23"/LConn1 -- 741/LConn1
  " kvar6"/LConn1 -- 722/RConn1
  " kvar15"/LConn3 -- 728/RConn3
  " kvar3"/LConn1 -- 712/LConn1
  " kvar9"/LConn2 -- 725/RConn2
  " kvar10"/LConn2 -- 720/RConn2
  " kvar9"/LConn1 -- 725/RConn1
  " kvar19"/LConn2 -- 735/RConn2
  " kvar19"/LConn3 -- 735/RConn3
  " kvar21"/LConn3 -- 737/RConn3
  " kvar8"/LConn2 -- 718/RConn2
  " kvar8"/LConn1 -- 718/RConn1
  " kvar16"/LConn3 -- 731/RConn3
  " kvar26"/LConn2 -- 732/LConn2
  " kvar26"/LConn1 -- 732/LConn1
  " kvar6"/LConn2 -- 722/RConn2
  " kvar27"/LConn1 -- 742/LConn1
  " kvar15"/LConn2 -- 728/RConn2
  " kvar16"/LConn1 -- 731/RConn1
  " kvar16"/LConn2 -- 731/RConn2
  " kvar3"/LConn3 -- 712/LConn3
  " kvar19"/LConn1 -- 735/RConn1
  " kvar24"/LConn1 -- 740/RConn1
  " kvar27"/LConn2 -- 742/LConn2
  " kvar23"/LConn2 -- 741/LConn2
  " kvar26"/LConn3 -- 732/LConn3
  " kvar23"/LConn3 -- 741/LConn3
  " kvar21"/LConn2 -- 737/RConn2
  SUBSTATION/RConn1 -- 799 - 701 Configuration 721/LConn1
  " kvar15"/LConn1 -- 728/RConn1
  " kvar11"/LConn3 -- 724/LConn3
  " kvar24"/LConn3 -- 740/RConn3
  " kvar10"/LConn3 -- 720/RConn3
  " kvar10"/LConn1 -- 720/RConn1
  " kvar27"/LConn3 -- 742/LConn3
  " kvar12"/LConn3 -- "744 - 729 config 724 "/LConn3
  " kvar21"/LConn1 -- 737/RConn1
  " kvar11"/LConn1 -- 724/LConn1
  " kvar24"/LConn2 -- 740/RConn2
  " kvar11"/LConn2 -- 724/LConn2
  " kvar12"/LConn2 -- "744 - 729 config 724 "/LConn2
  " kvar12"/LConn1 -- "744 - 729 config 724 "/LConn1

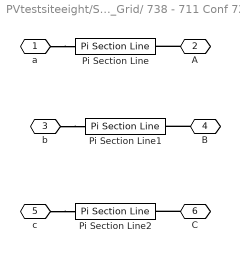
== system PVtestsiteeight/SS_Grid/ 738 - 711 Conf 723  ==
  Pi Section Line : powerlib/Elements/Pi Section Line  LConnTagsString=__new0  RConnTagsString=__new0  Frequency=60  Resistance=0.803807  Inductance=0.0011064  Capacitance=1.23355e-07  Length=D  PiSections=1  Measurements=None
      settings: AttributesFormatString=\n  SourceProductBaseCode=PS
  Pi Section Line1 : powerlib/Elements/Pi Section Line  LConnTagsString=__new0  RConnTagsString=__new0  Frequency=60  Resistance=0.80915157  Inductance=0.00104267  Capacitance=1.233552e-07  Length=D  PiSections=1  Measurements=None
      settings: AttributesFormatString=\n  SourceProductBaseCode=PS
  Pi Section Line2 : powerlib/Elements/Pi Section Line  LConnTagsString=__new0  RConnTagsString=__new0  Frequency=60  Resistance=0.8038077  Inductance=0.0011064  Capacitance=1.23355e-07  Length=D  PiSections=1  Measurements=None
      settings: AttributesFormatString=\n  SourceProductBaseCode=PS
  a : PMIOPort  Side=Left
  A : PMIOPort  Port=2  Side=Right
  b : PMIOPort  Port=3  Side=Left
  B : PMIOPort  Port=4  Side=Right
  c : PMIOPort  Port=5  Side=Left
  C : PMIOPort  Port=6  Side=Right
  connections:
  a/RConn1 -- Pi Section Line/LConn1
  A/RConn1 -- Pi Section Line/RConn1
  b/RConn1 -- Pi Section Line1/LConn1
  B/RConn1 -- Pi Section Line1/RConn1
  c/RConn1 -- Pi Section Line2/LConn1
  C/RConn1 -- Pi Section Line2/RConn1

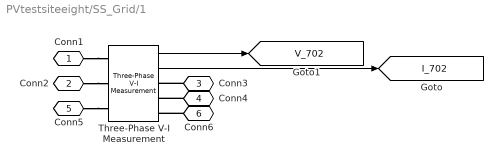
== system PVtestsiteeight/SS_Grid/1 ==
  Three-Phase V-I Measurement : powerlib/Measurements/Three-Phase V-I Measurement  VoltageMeasurement=phase-to-ground  SetLabelV=off  LabelV=Vabc  Vpu=off  VpuLL=off  CurrentMeasurement=yes  SetLabelI=off  LabelI=Iabc  Ipu=off  Pbase=100e6  Vbase=500e3  OutputType=Complex  PhasorSimulation=off  PSBequivalent=0
  Conn1 : PMIOPort  Side=Left
  Conn2 : PMIOPort  Port=2  Side=Left
  Conn3 : PMIOPort  Port=3  Side=Right
  Conn4 : PMIOPort  Port=4  Side=Right
  Conn5 : PMIOPort  Port=5  Side=Left
  Conn6 : PMIOPort  Port=6  Side=Right
  tag scope: I_702=global, V_702=global
  wires:
  Three-Phase V-I Measurement/1 -> [V_702]
  Three-Phase V-I Measurement/2 -> [I_702]
  connections:
  Conn1/RConn1 -- Three-Phase V-I Measurement/LConn1
  Conn2/RConn1 -- Three-Phase V-I Measurement/LConn2
  Conn3/RConn1 -- Three-Phase V-I Measurement/RConn1
  Conn4/RConn1 -- Three-Phase V-I Measurement/RConn2
  Conn5/RConn1 -- Three-Phase V-I Measurement/LConn3
  Conn6/RConn1 -- Three-Phase V-I Measurement/RConn3

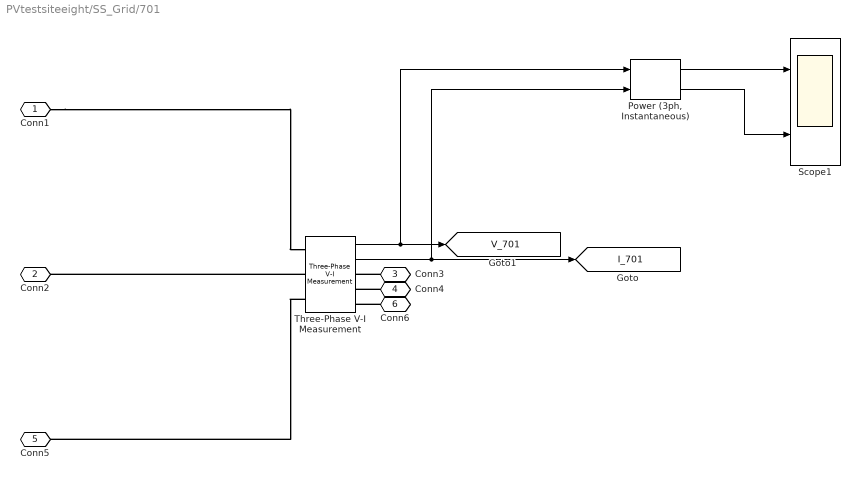
== system PVtestsiteeight/SS_Grid/701 ==
  "Power (3ph, Instantaneous)" : powerlib_meascontrol/Measurements/Power (3ph, Instantaneous)
  Scope1 : Scope  NumInputPorts=2
  Three-Phase V-I Measurement : powerlib/Measurements/Three-Phase V-I Measurement  VoltageMeasurement=phase-to-ground  SetLabelV=off  LabelV=Vabc  Vpu=off  VpuLL=off  CurrentMeasurement=yes  SetLabelI=off  LabelI=Iabc  Ipu=off  Pbase=100e6  Vbase=500e3  OutputType=Complex  PhasorSimulation=off  PSBequivalent=0
  Conn1 : PMIOPort  Side=Left
  Conn2 : PMIOPort  Port=2  Side=Left
  Conn3 : PMIOPort  Port=3  Side=Right
  Conn4 : PMIOPort  Port=4  Side=Right
  Conn5 : PMIOPort  Port=5  Side=Left
  Conn6 : PMIOPort  Port=6  Side=Right
  tag scope: I_701=global, V_701=global
  wires:
  Three-Phase V-I Measurement/2 -> "Power (3ph, Instantaneous)"/2, [I_701]
  Three-Phase V-I Measurement/1 -> "Power (3ph, Instantaneous)"/1, [V_701]
  "Power (3ph, Instantaneous)"/1 -> Scope1/1
  "Power (3ph, Instantaneous)"/2 -> Scope1/2
  connections:
  Conn6/RConn1 -- Three-Phase V-I Measurement/RConn3
  Three-Phase V-I Measurement/LConn3 -- Conn5/RConn1
  Conn4/RConn1 -- Three-Phase V-I Measurement/RConn2
  Conn3/RConn1 -- Three-Phase V-I Measurement/RConn1
  Three-Phase V-I Measurement/LConn2 -- Conn2/RConn1
  Conn1/RConn1 -- Three-Phase V-I Measurement/LConn1

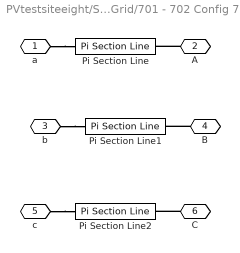
== system PVtestsiteeight/SS_Grid/701 - 702 Config 722 ==
  Pi Section Line : powerlib/Elements/Pi Section Line  LConnTagsString=__new0  RConnTagsString=__new0  Frequency=60  Resistance=0.2952141  Inductance=0.0004900224  Capacitance=2.10695e-07  Length=D  PiSections=1  Measurements=None
      settings: AttributesFormatString=\n  SourceProductBaseCode=PS
  Pi Section Line1 : powerlib/Elements/Pi Section Line  LConnTagsString=__new0  RConnTagsString=__new0  Frequency=60  Resistance=0.27887208  Inductance=0.0004413993  Capacitance=2.10695e-07  Length=D  PiSections=1  Measurements=None
      settings: AttributesFormatString=\n  SourceProductBaseCode=PS
  Pi Section Line2 : powerlib/Elements/Pi Section Line  LConnTagsString=__new0  RConnTagsString=__new0  Frequency=60  Resistance=0.29521418  Inductance=0.00049002245  Capacitance=2.106958e-07  Length=D  PiSections=1  Measurements=None
      settings: AttributesFormatString=\n  SourceProductBaseCode=PS
  a : PMIOPort  Side=Left
  A : PMIOPort  Port=2  Side=Right
  b : PMIOPort  Port=3  Side=Left
  B : PMIOPort  Port=4  Side=Right
  c : PMIOPort  Port=5  Side=Left
  C : PMIOPort  Port=6  Side=Right
  connections:
  C/RConn1 -- Pi Section Line2/RConn1
  c/RConn1 -- Pi Section Line2/LConn1
  B/RConn1 -- Pi Section Line1/RConn1
  b/RConn1 -- Pi Section Line1/LConn1
  A/RConn1 -- Pi Section Line/RConn1
  a/RConn1 -- Pi Section Line/LConn1

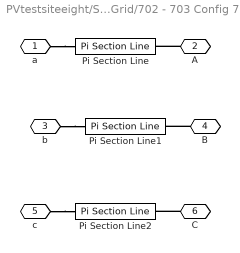
== system PVtestsiteeight/SS_Grid/702 - 703 Config 722 ==
  Pi Section Line : powerlib/Elements/Pi Section Line  LConnTagsString=__new0  RConnTagsString=__new0  Frequency=60  Resistance=0.2952141  Inductance=0.0004900224  Capacitance=2.10695e-07  Length=D  PiSections=1  Measurements=None
      settings: AttributesFormatString=\n  SourceProductBaseCode=PS
  Pi Section Line1 : powerlib/Elements/Pi Section Line  LConnTagsString=__new0  RConnTagsString=__new0  Frequency=60  Resistance=0.27887208  Inductance=0.0004413993  Capacitance=2.10695e-07  Length=D  PiSections=1  Measurements=None
      settings: AttributesFormatString=\n  SourceProductBaseCode=PS
  Pi Section Line2 : powerlib/Elements/Pi Section Line  LConnTagsString=__new0  RConnTagsString=__new0  Frequency=60  Resistance=0.29521418  Inductance=0.00049002245  Capacitance=2.106958e-07  Length=D  PiSections=1  Measurements=None
      settings: AttributesFormatString=\n  SourceProductBaseCode=PS
  a : PMIOPort  Side=Left
  A : PMIOPort  Port=2  Side=Right
  b : PMIOPort  Port=3  Side=Left
  B : PMIOPort  Port=4  Side=Right
  c : PMIOPort  Port=5  Side=Left
  C : PMIOPort  Port=6  Side=Right
  connections:
  a/RConn1 -- Pi Section Line/LConn1
  A/RConn1 -- Pi Section Line/RConn1
  b/RConn1 -- Pi Section Line1/LConn1
  B/RConn1 -- Pi Section Line1/RConn1
  c/RConn1 -- Pi Section Line2/LConn1
  C/RConn1 -- Pi Section Line2/RConn1

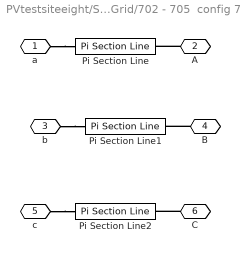
== system PVtestsiteeight/SS_Grid/702 - 705  config 724  ==
  Pi Section Line : powerlib/Elements/Pi Section Line  LConnTagsString=__new0  RConnTagsString=__new0  Frequency=60  Resistance=1.3019001  Inductance=0.0012787  Capacitance=9.93038e-08  Length=D  PiSections=1  Measurements=None
      settings: AttributesFormatString=\n  SourceProductBaseCode=PS
  Pi Section Line1 : powerlib/Elements/Pi Section Line  LConnTagsString=__new0  RConnTagsString=__new0  Frequency=60  Resistance=1.309108  Inductance=0.001219369  Capacitance=9.9303e-08  Length=D  PiSections=1  Measurements=None
      settings: AttributesFormatString=\n  SourceProductBaseCode=PS
  Pi Section Line2 : powerlib/Elements/Pi Section Line  LConnTagsString=__new0  RConnTagsString=__new0  Frequency=60  Resistance=1.3019001  Inductance=0.0012787  Capacitance=9.93038e-08  Length=D  PiSections=1  Measurements=None
      settings: AttributesFormatString=\n  SourceProductBaseCode=PS
  a : PMIOPort  Side=Left
  A : PMIOPort  Port=2  Side=Right
  b : PMIOPort  Port=3  Side=Left
  B : PMIOPort  Port=4  Side=Right
  c : PMIOPort  Port=5  Side=Left
  C : PMIOPort  Port=6  Side=Right
  connections:
  C/RConn1 -- Pi Section Line2/RConn1
  c/RConn1 -- Pi Section Line2/LConn1
  B/RConn1 -- Pi Section Line1/RConn1
  b/RConn1 -- Pi Section Line1/LConn1
  A/RConn1 -- Pi Section Line/RConn1
  a/RConn1 -- Pi Section Line/LConn1

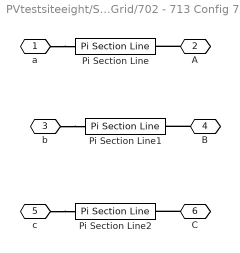
== system PVtestsiteeight/SS_Grid/702 - 713 Config 723 ==
  Pi Section Line : powerlib/Elements/Pi Section Line  LConnTagsString=__new0  RConnTagsString=__new0  Frequency=60  Resistance=0.803807  Inductance=0.0011064  Capacitance=1.23355e-07  Length=D  PiSections=1  Measurements=None
      settings: AttributesFormatString=\n  SourceProductBaseCode=PS
  Pi Section Line1 : powerlib/Elements/Pi Section Line  LConnTagsString=__new0  RConnTagsString=__new0  Frequency=60  Resistance=0.80915157  Inductance=0.00104267  Capacitance=1.233552e-07  Length=D  PiSections=1  Measurements=None
      settings: AttributesFormatString=\n  SourceProductBaseCode=PS
  Pi Section Line2 : powerlib/Elements/Pi Section Line  LConnTagsString=__new0  RConnTagsString=__new0  Frequency=60  Resistance=0.8038077  Inductance=0.0011064  Capacitance=1.23355e-07  Length=D  PiSections=1  Measurements=None
      settings: AttributesFormatString=\n  SourceProductBaseCode=PS
  a : PMIOPort  Side=Left
  A : PMIOPort  Port=2  Side=Right
  b : PMIOPort  Port=3  Side=Left
  B : PMIOPort  Port=4  Side=Right
  c : PMIOPort  Port=5  Side=Left
  C : PMIOPort  Port=6  Side=Right
  connections:
  a/RConn1 -- Pi Section Line/LConn1
  A/RConn1 -- Pi Section Line/RConn1
  b/RConn1 -- Pi Section Line1/LConn1
  B/RConn1 -- Pi Section Line1/RConn1
  c/RConn1 -- Pi Section Line2/LConn1
  C/RConn1 -- Pi Section Line2/RConn1

== system PVtestsiteeight/SS_Grid/703 ==
  Three-Phase V-I Measurement : powerlib/Measurements/Three-Phase V-I Measurement  VoltageMeasurement=phase-to-ground  SetLabelV=off  LabelV=Vabc  Vpu=off  VpuLL=off  CurrentMeasurement=yes  SetLabelI=off  LabelI=Iabc  Ipu=off  Pbase=100e6  Vbase=500e3  OutputType=Complex  PhasorSimulation=off  PSBequivalent=0
  Conn1 : PMIOPort  Side=Left
  Conn2 : PMIOPort  Port=2  Side=Left
  Conn3 : PMIOPort  Port=3  Side=Right
  Conn4 : PMIOPort  Port=4  Side=Right
  Conn5 : PMIOPort  Port=5  Side=Left
  Conn6 : PMIOPort  Port=6  Side=Right
  tag scope: I_703=global, V_703=global
  wires:
  Three-Phase V-I Measurement/2 -> [I_703]
  Three-Phase V-I Measurement/1 -> [V_703]
  connections:
  Conn6/RConn1 -- Three-Phase V-I Measurement/RConn3
  Conn5/RConn1 -- Three-Phase V-I Measurement/LConn3
  Conn4/RConn1 -- Three-Phase V-I Measurement/RConn2
  Conn3/RConn1 -- Three-Phase V-I Measurement/RConn1
  Conn2/RConn1 -- Three-Phase V-I Measurement/LConn2
  Conn1/RConn1 -- Three-Phase V-I Measurement/LConn1

== system PVtestsiteeight/SS_Grid/703 - 727 config 724 ==
  Pi Section Line : powerlib/Elements/Pi Section Line  LConnTagsString=__new0  RConnTagsString=__new0  Frequency=60  Resistance=1.3019001  Inductance=0.0012787  Capacitance=9.93038e-08  Length=D  PiSections=1  Measurements=None
      settings: AttributesFormatString=\n  SourceProductBaseCode=PS
  Pi Section Line1 : powerlib/Elements/Pi Section Line  LConnTagsString=__new0  RConnTagsString=__new0  Frequency=60  Resistance=1.309108  Inductance=0.001219369  Capacitance=9.9303e-08  Length=D  PiSections=1  Measurements=None
      settings: AttributesFormatString=\n  SourceProductBaseCode=PS
  Pi Section Line2 : powerlib/Elements/Pi Section Line  LConnTagsString=__new0  RConnTagsString=__new0  Frequency=60  Resistance=1.3019001  Inductance=0.0012787  Capacitance=9.93038e-08  Length=D  PiSections=1  Measurements=None
      settings: AttributesFormatString=\n  SourceProductBaseCode=PS
  a : PMIOPort  Side=Left
  A : PMIOPort  Port=2  Side=Right
  b : PMIOPort  Port=3  Side=Left
  B : PMIOPort  Port=4  Side=Right
  c : PMIOPort  Port=5  Side=Left
  C : PMIOPort  Port=6  Side=Right
  connections:
  a/RConn1 -- Pi Section Line/LConn1
  A/RConn1 -- Pi Section Line/RConn1
  b/RConn1 -- Pi Section Line1/LConn1
  B/RConn1 -- Pi Section Line1/RConn1
  c/RConn1 -- Pi Section Line2/LConn1
  C/RConn1 -- Pi Section Line2/RConn1

== system PVtestsiteeight/SS_Grid/703 - 730 Config 723 ==
  Pi Section Line : powerlib/Elements/Pi Section Line  LConnTagsString=__new0  RConnTagsString=__new0  Frequency=60  Resistance=0.803807  Inductance=0.0011064  Capacitance=1.23355e-07  Length=D  PiSections=1  Measurements=None
      settings: AttributesFormatString=\n  SourceProductBaseCode=PS
  Pi Section Line1 : powerlib/Elements/Pi Section Line  LConnTagsString=__new0  RConnTagsString=__new0  Frequency=60  Resistance=0.80915157  Inductance=0.00104267  Capacitance=1.233552e-07  Length=D  PiSections=1  Measurements=None
      settings: AttributesFormatString=\n  SourceProductBaseCode=PS
  Pi Section Line2 : powerlib/Elements/Pi Section Line  LConnTagsString=__new0  RConnTagsString=__new0  Frequency=60  Resistance=0.8038077  Inductance=0.0011064  Capacitance=1.23355e-07  Length=D  PiSections=1  Measurements=None
      settings: AttributesFormatString=\n  SourceProductBaseCode=PS
  a : PMIOPort  Side=Left
  A : PMIOPort  Port=2  Side=Right
  b : PMIOPort  Port=3  Side=Left
  B : PMIOPort  Port=4  Side=Right
  c : PMIOPort  Port=5  Side=Left
  C : PMIOPort  Port=6  Side=Right
  connections:
  C/RConn1 -- Pi Section Line2/RConn1
  c/RConn1 -- Pi Section Line2/LConn1
  B/RConn1 -- Pi Section Line1/RConn1
  b/RConn1 -- Pi Section Line1/LConn1
  A/RConn1 -- Pi Section Line/RConn1
  a/RConn1 -- Pi Section Line/LConn1

== system PVtestsiteeight/SS_Grid/704 ==
  Three-Phase V-I Measurement : powerlib/Measurements/Three-Phase V-I Measurement  VoltageMeasurement=phase-to-ground  SetLabelV=off  LabelV=Vabc  Vpu=off  VpuLL=off  CurrentMeasurement=yes  SetLabelI=off  LabelI=Iabc  Ipu=off  Pbase=100e6  Vbase=500e3  OutputType=Complex  PhasorSimulation=off  PSBequivalent=0
  Conn1 : PMIOPort  Side=Left
  Conn2 : PMIOPort  Port=2  Side=Left
  Conn3 : PMIOPort  Port=3  Side=Right
  Conn4 : PMIOPort  Port=4  Side=Right
  Conn5 : PMIOPort  Port=5  Side=Left
  Conn6 : PMIOPort  Port=6  Side=Right
  tag scope: I_704=global, V_704=global
  wires:
  Three-Phase V-I Measurement/2 -> [I_704]
  Three-Phase V-I Measurement/1 -> [V_704]
  connections:
  Conn6/RConn1 -- Three-Phase V-I Measurement/RConn3
  Conn5/RConn1 -- Three-Phase V-I Measurement/LConn3
  Conn4/RConn1 -- Three-Phase V-I Measurement/RConn2
  Conn3/RConn1 -- Three-Phase V-I Measurement/RConn1
  Conn2/RConn1 -- Three-Phase V-I Measurement/LConn2
  Conn1/RConn1 -- Three-Phase V-I Measurement/LConn1

== system PVtestsiteeight/SS_Grid/704 - 714 config 724 ==
  Pi Section Line : powerlib/Elements/Pi Section Line  LConnTagsString=__new0  RConnTagsString=__new0  Frequency=60  Resistance=1.3019001  Inductance=0.0012787  Capacitance=9.93038e-08  Length=D  PiSections=1  Measurements=None
      settings: AttributesFormatString=\n  SourceProductBaseCode=PS
  Pi Section Line1 : powerlib/Elements/Pi Section Line  LConnTagsString=__new0  RConnTagsString=__new0  Frequency=60  Resistance=1.309108  Inductance=0.001219369  Capacitance=9.9303e-08  Length=D  PiSections=1  Measurements=None
      settings: AttributesFormatString=\n  SourceProductBaseCode=PS
  Pi Section Line2 : powerlib/Elements/Pi Section Line  LConnTagsString=__new0  RConnTagsString=__new0  Frequency=60  Resistance=1.3019001  Inductance=0.0012787  Capacitance=9.93038e-08  Length=D  PiSections=1  Measurements=None
      settings: AttributesFormatString=\n  SourceProductBaseCode=PS
  a : PMIOPort  Side=Left
  A : PMIOPort  Port=2  Side=Right
  b : PMIOPort  Port=3  Side=Left
  B : PMIOPort  Port=4  Side=Right
  c : PMIOPort  Port=5  Side=Left
  C : PMIOPort  Port=6  Side=Right
  connections:
  C/RConn1 -- Pi Section Line2/RConn1
  c/RConn1 -- Pi Section Line2/LConn1
  B/RConn1 -- Pi Section Line1/RConn1
  b/RConn1 -- Pi Section Line1/LConn1
  A/RConn1 -- Pi Section Line/RConn1
  a/RConn1 -- Pi Section Line/LConn1
